simulink model "lab1"  (R2023b)
settings: Solver=VariableStepAuto  StartTime=0.0  StopTime=10.0  RelTol=1e-3
settings Model: Creator=DELL  LastModifiedBy=DELL

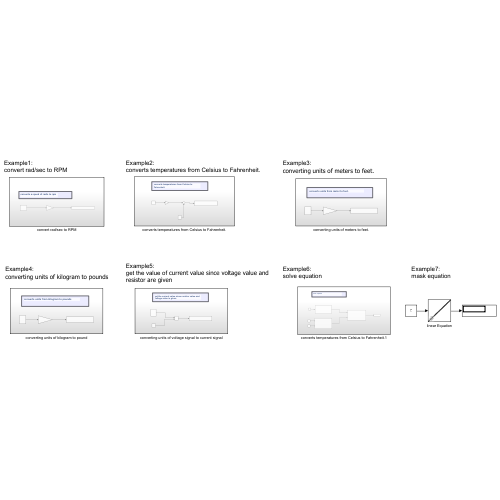
[thumbnail: Simulink's stored preview of the top-level diagram]
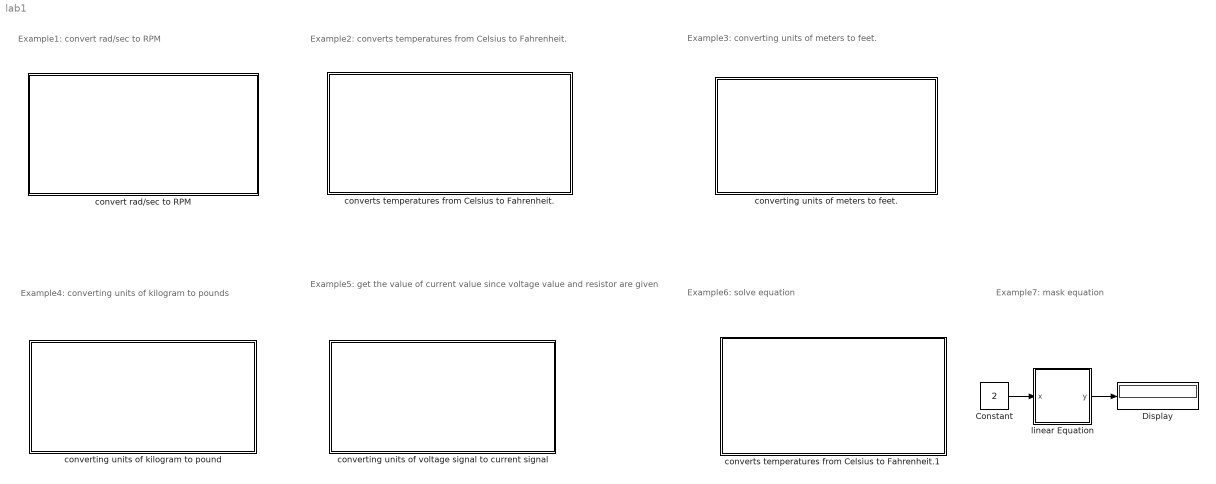
== system lab1 ==
  note: Example2:
      | converts temperatures from Celsius to Fahrenheit.
  note: Example1:
      | convert rad/sec to RPM
  note: Example3:
      | converting units of meters to feet.
  note: Example4:
      | converting units of kilogram to pounds
  note: Example5:
      | get the value of current value since voltage value and resistor are given
  note: Example6:
      | solve equation
  note: Example7:
      | mask equation
  Constant : Constant  Value=2
  Display : Display
  convert rad/sec to RPM : Subsystem
  converting units of kilogram to pound : Subsystem
  converting units of meters to feet. : Subsystem
  converting units of voltage signal to current signal : Subsystem
  converts temperatures from Celsius to Fahrenheit. : Subsystem
  converts temperatures from Celsius to Fahrenheit.1 : Subsystem
  linear Equation : Subsystem  mask{m=2, c=2}
      mask prompts: m "slope"; c "constant"
      mask Display:
      | x=linspace(0,1,101);
      | t=linspace(0,1,101);
      | 
      | plot(x,t);
  wires:
  Constant/1 -> linear Equation/1(x)
  linear Equation/1(y) -> Display/1

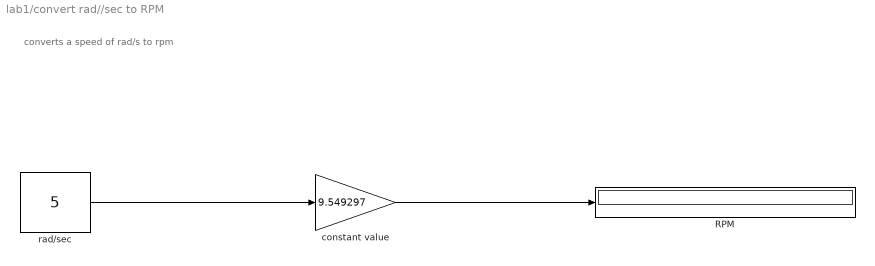
== system lab1/convert rad//sec to RPM ==
  note: converts a speed of rad/s to rpm
  RPM : Display
      settings: Decimation=5
  constant value : Gain  Gain=9.549297
  rad/sec : Constant  Value=5
  wires:
  constant value/1 -> RPM/1
  rad/sec/1 -> constant value/1

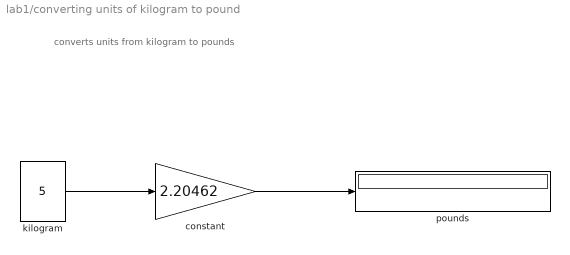
== system lab1/converting units of kilogram to pound ==
  note: converts units from kilogram to pounds
  "constant " : Gain  Gain=2.20462
  kilogram : Constant  Value=5
  pounds : Display
  wires:
  kilogram/1 -> "constant "/1
  "constant "/1 -> pounds/1

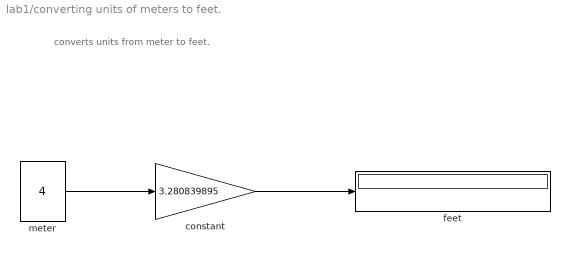
== system lab1/converting units of meters to feet. ==
  note: converts units from meter to feet.
  "constant " : Gain  Gain=3.280839895
  feet : Display
  meter : Constant  Value=4
  wires:
  meter/1 -> "constant "/1
  "constant "/1 -> feet/1

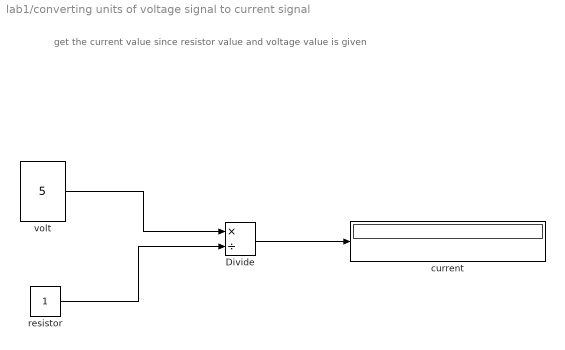
== system lab1/converting units of voltage signal to current signal ==
  note: get the current value since resistor value and voltage value is given
  Divide : Product  Inputs=*/
  "current " : Display
  resistor : Constant
  volt : Constant  Value=5
  wires:
  volt/1 -> Divide/1
  resistor/1 -> Divide/2
  Divide/1 -> "current "/1

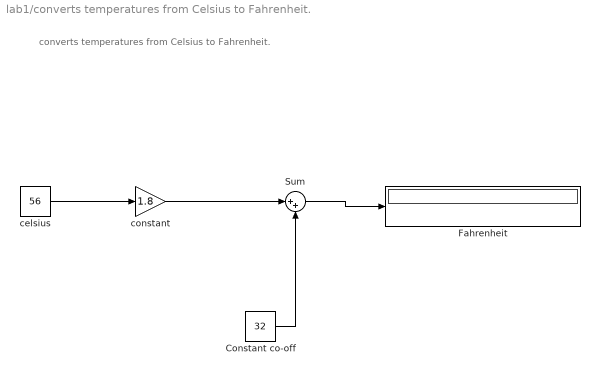
== system lab1/converts temperatures from Celsius to Fahrenheit. ==
  note: converts temperatures from Celsius to Fahrenheit.
  Constant co-off : Constant  Value=32
  Fahrenheit : Display
  Sum : Sum  Inputs=|++
  celsius : Constant  Value=56
  "constant " : Gain  Gain=1.8
  wires:
  celsius/1 -> "constant "/1
  "constant "/1 -> Sum/1
  Constant co-off/1 -> Sum/2
  Sum/1 -> Fahrenheit/1

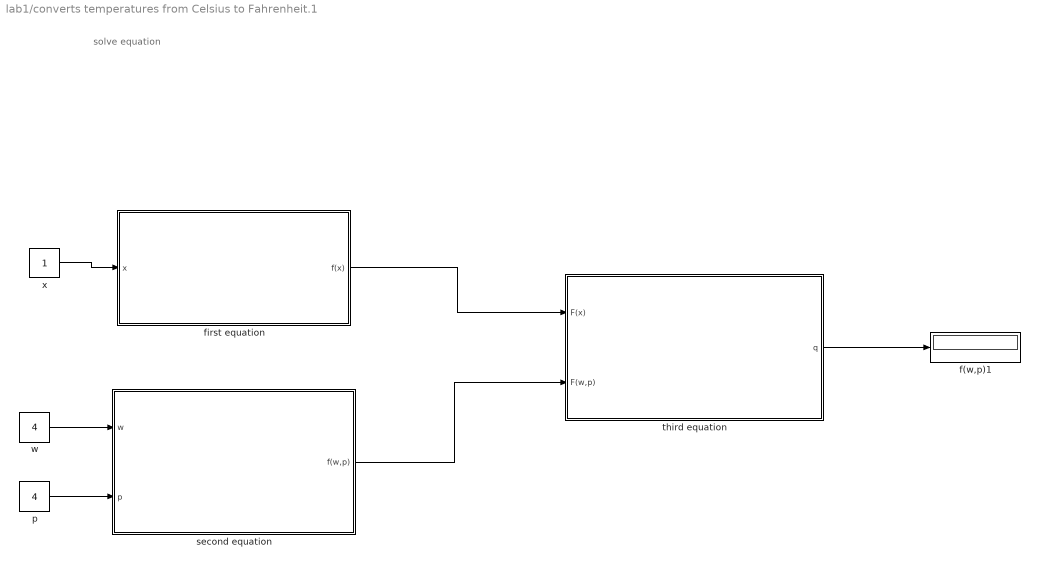
== system lab1/converts temperatures from Celsius to Fahrenheit.1 ==
  note: solve equation
  f(w,p)1 : Display
  first equation : Subsystem
  p : Constant  Value=4
  "second equation " : Subsystem
  third equation : Subsystem
  w : Constant  Value=4
  x : Constant
  wires:
  x/1 -> first equation/1(x)
  first equation/1(f(x)) -> third equation/1(F(x))
  w/1 -> "second equation "/1(w)
  p/1 -> "second equation "/2(p)
  "second equation "/1(f(w,p)) -> third equation/2(F(w,p))
  third equation/1(q) -> f(w,p)1/1

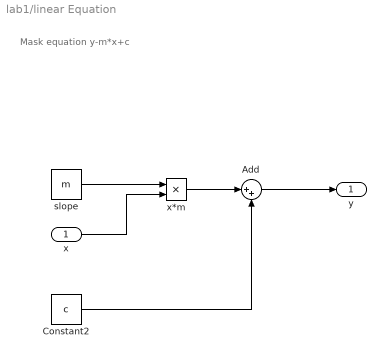
== system lab1/linear Equation ==
  note: Mask equation
      | y-m*x+c
  x : Inport
  Add : Sum  Inputs=|++
  Constant2 : Constant  Value=c
  slope : Constant  Value=m
  x*m : Product
  y : Outport
  wires:
  slope/1 -> x*m/1
  x/1 -> x*m/2
  x*m/1 -> Add/1
  Constant2/1 -> Add/2
  Add/1 -> y/1

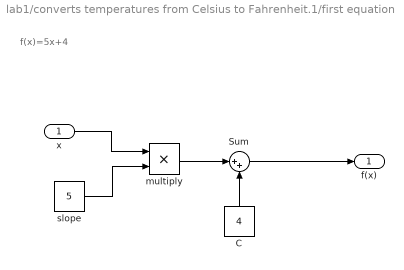
== system lab1/converts temperatures from Celsius to Fahrenheit.1/first equation ==
  note: f(x)=5x+4
  x : Inport
  C : Constant  Value=4
  Sum : Sum  Inputs=|++
  multiply : Product
  slope : Constant  Value=5
  f(x) : Outport
  wires:
  Sum/1 -> f(x)/1
  C/1 -> Sum/2
  x/1 -> multiply/1
  multiply/1 -> Sum/1
  slope/1 -> multiply/2

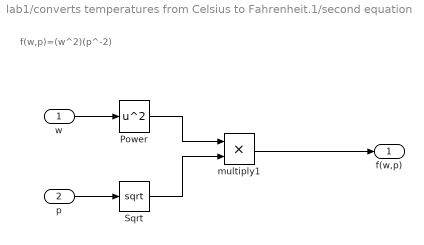
== system lab1/converts temperatures from Celsius to Fahrenheit.1/second equation  ==
  note: f(w,p)=(w^2)(p^-2)
  w : Inport
  p : Inport  Port=2
  Power : Math  Operator=square
  Sqrt : Sqrt
  multiply1 : Product
  f(w,p) : Outport
  wires:
  multiply1/1 -> f(w,p)/1
  Power/1 -> multiply1/1
  p/1 -> Sqrt/1
  Sqrt/1 -> multiply1/2
  w/1 -> Power/1

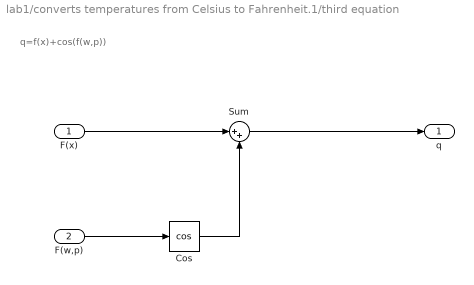
== system lab1/converts temperatures from Celsius to Fahrenheit.1/third equation ==
  note: q=f(x)+cos(f(w,p))
  F(x) : Inport
  F(w,p) : Inport  Port=2
  Cos : Trigonometry  Operator=cos
  Sum : Sum  Inputs=|++
  q : Outport
  wires:
  F(w,p)/1 -> Cos/1
  F(x)/1 -> Sum/1
  Cos/1 -> Sum/2
  Sum/1 -> q/1
